simulink model "chap11_3sim"  (R2015a)
settings: Solver=ode45  StartTime=0.0  StopTime=3  RelTol=1e-3
settings Model: Creator=zhr  LastModifiedBy=IT

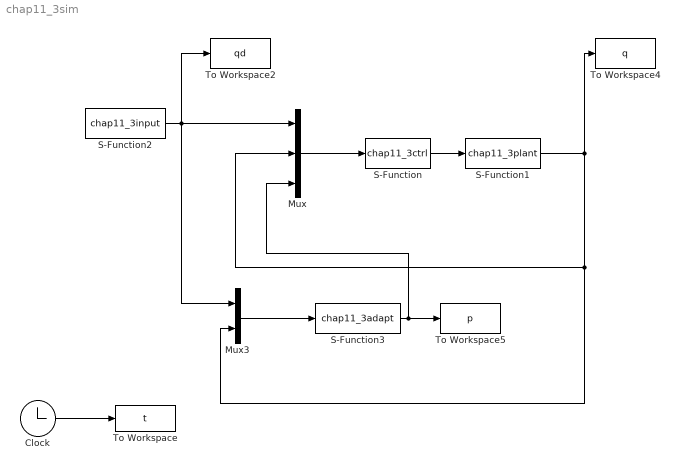
== system chap11_3sim ==
  Clock : Clock
  Mux : Mux  Inputs=3
  Mux3 : Mux  Inputs=2
  S-Function : S-Function  FunctionName=chap11_3ctrl
  S-Function1 : S-Function  FunctionName=chap11_3plant
  S-Function2 : S-Function  FunctionName=chap11_3input
  S-Function3 : S-Function  FunctionName=chap11_3adapt
  To Workspace : ToWorkspace  VariableName=t  SampleTime=-1
  To Workspace2 : ToWorkspace  VariableName=qd  SampleTime=-1
  To Workspace4 : ToWorkspace  VariableName=q  SampleTime=-1
  To Workspace5 : ToWorkspace  VariableName=p  SampleTime=-1
  wires:
  Clock/1 -> To Workspace/1
  Mux/1 -> S-Function/1
  S-Function/1 -> S-Function1/1
  S-Function1/1 -> Mux/2, Mux3/2, To Workspace4/1
  S-Function2/1 -> Mux3/1, To Workspace2/1, Mux/1
  S-Function3/1 -> To Workspace5/1, Mux/3
  Mux3/1 -> S-Function3/1
